simulink model "NarmaMotorS444"  (R2019b)
settings: Solver=FixedStepAuto  StartTime=0.0  StopTime=30  FixedStep=0.001  RelTol=1e-3
libraries: neural x1, simulink x1
settings Model: Creator=Emanuel  LastModifiedBy=Emanuel

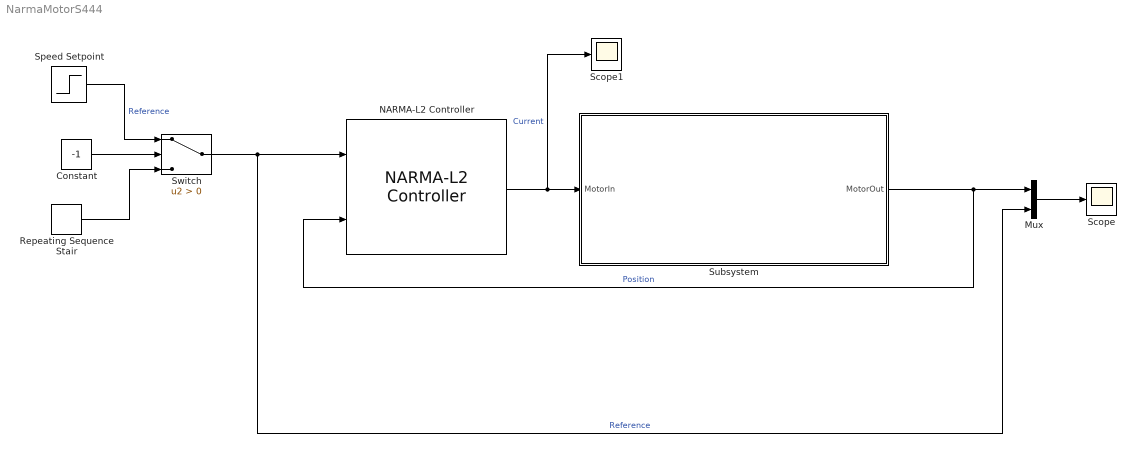
== system NarmaMotorS444 ==
  Constant : Constant  Value=-1
  Mux : Mux  Inputs=2
  NARMA-L2 Controller : neural/Control Systems/NARMA-L2 Controller  Normalize=0  IW1_1=[-0.00010236025899872490809 2.7586514069221412045e-05 -1.0105911937399750936e-05 1.3256012738340794443e-05 -0.00012177307341552546399 9.4877524383052964214e-05 0.00016811599685202734166;-0.9314764402798860754 -4.0881413596783540143 -1.7151050991711540572 4.9130010420420884287 -1.2247909630343454257 -2.4839816062380393191 -2.4615143768260137058;-9.4112593425783597212 6.7702586754591775886 5.1048148087375526671 -4.0293352992265125678 -1.5860815268788490684 -2.0648737785344812856 1.8072837448183800557;-6.6517733281320357008 -0.39174207719143561146 4.2930162877030273449 5.6049907770564697529 -0.78433332140491096585 -0.37768508077910345477 -0.42004150889728419926]  IW3_2=[-1.1884782210932853808 -2.6026502224083305492 0.77838373361354451507 2.7173822538084015932 -0.25745108287285101145 -0.020471196678414908116 -0.46445815351973612772;-0.25444398603368395539 0.30008368263429602285 -0.0074376747696380850552 0.59158184449179707087 0.34380512952139080651 -0.87996185058892895103 1.4365647591299173236;0.077286965668154586351 0.15379022274742931709 0.49370556823373967781 -0.72901144987097687977 -6.3829467961491106465 -24.779081553654108916 7.8291606863920542025;0.60195820662206900309 -2.4802125107952845973 -2.0779594279619324482 4.3693209146217668604 0.97906627286878922245 -0.91348821354353892943 0.52582308602693783595]  IW5_3=2.791472264992422847  LW2_1=[-116.75369921671634188 -15.359712959372973984 -10.101511034971979441 14.81434611829450354]  LW4_3=[-1.5956321863719566956 2.5213572345198809188 2.7013939494135672525 0.99504426028142600735]  LW5_4=-0.13241264861201840208  LW6_5=-3.346419847725022656  LW6_2=119.28421133069207372  B1=[0.47304643530334977708;0.069176646723712875708;-2.1542505763216901471;1.1374465832201940962]  B2=14.49636392954983144  B3=[1.2607629848186907573;0.0297410068321030778;3.2197369295363471586;0.27292507888832240326]  B4=2.1680736346604891907  Limit_output=0  min_output=-Inf  max_output=Inf  Use_Previous_Weights=1  Ts=0.05  S1=4  Ni=4  Nj=4  sim_file=SoleModelNoDistrubance  trainfun=trainlm  Use_validation=1  Use_Testing=1  max_i=40  min_i=1  max_i_int=4  min_i_int=2  sam_training=10000  epochs=500  minp=1.2838861864609374397  maxp=39.753006491435613157  mint=2000.3866487334141766  maxt=39.753006491435613157
      settings: SourceProductName=Deep Learning Toolbox  SourceProductBaseCode=NN
  Repeating Sequence Stair : simulink/Sources/Repeating Sequence Stair  OutValues=[1000 2000 3000 4000 5000].'  tsamp=4  OutMin=[]  OutMax=[]  OutDataTypeStr=double  OutputDataTypeScalingMode=double  OutDataType=fixdt(0,8)  ConRadixGroup=Best Precision: Vector-wise  OutScaling=2^-12
  Scope : Scope
  Scope1 : Scope
  Speed Setpoint : Step  Time=5  Before=2000  After=3000  SampleTime=0
  Subsystem : Subsystem
  Switch : Switch  Criteria=u2 > Threshold
  wires:
  NARMA-L2 Controller/1 -> Scope1/1, Subsystem/1(MotorIn)  "Current"
  Subsystem/1("MotorOut ") -> NARMA-L2 Controller/2, Mux/1  "Position"
  Mux/1 -> Scope/1
  Switch/1 -> Mux/2, NARMA-L2 Controller/1  "Reference"
  Repeating Sequence Stair/1 -> Switch/3
  Speed Setpoint/1 -> Switch/1  "Reference"
  Constant/1 -> Switch/2

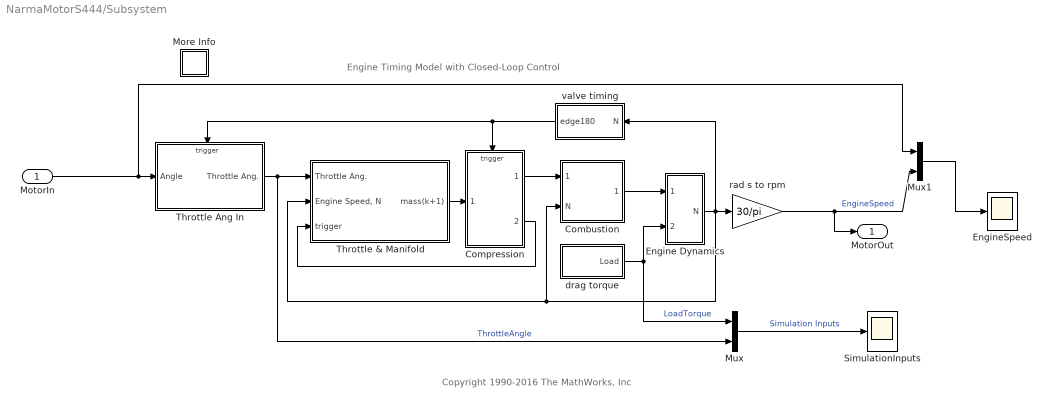
== system NarmaMotorS444/Subsystem ==
  note: Copyright 1990-2016 The MathWorks, Inc
  note: Engine Timing Model with Closed-Loop Control
  MotorIn : Inport
  Combustion : Subsystem
  Compression : Subsystem  TreatAsAtomicUnit=on
  Engine Dynamics : Subsystem
  EngineSpeed : Scope
  More Info : Subsystem
      settings: OpenFcn=showdemo(bdroot(gcb))
      mask Display: disp('?')
  Mux : Mux  Inputs=2
  Mux1 : Mux  Inputs=2
  SimulationInputs : Scope
  Throttle & Manifold : Subsystem
  Throttle Ang In : Subsystem  TreatAsAtomicUnit=on
  drag torque : Subsystem
  rad s to rpm : Gain  Gain=30/pi  SaturateOnIntegerOverflow=on  OutDataTypeStr=Inherit: Same as input  ParamDataTypeStr=Inherit: Same as input
  valve timing : Subsystem
  "MotorOut " : Outport
  wires:
  Combustion/1(Torque) -> Engine Dynamics/1(Teng)
  Throttle Ang In/1(Throttle Ang.) -> Mux/2, Throttle & Manifold/1(Throttle Ang.)  "ThrottleAngle"
  drag torque/1(Load) -> Mux/1, Engine Dynamics/2(Tload)  "LoadTorque"
  MotorIn/1 -> Mux1/1, Throttle Ang In/1(Angle)
  Throttle & Manifold/1(mass(k+1)) -> Compression/1(mass(k+1))
  Compression/2(trigger) -> Throttle & Manifold/3(trigger)
  Mux/1 -> SimulationInputs/1  "Simulation Inputs"
  rad s to rpm/1 -> "MotorOut "/1, Mux1/2  "EngineSpeed"
  Compression/1(mass(k)) -> Combustion/1(Air Charge)
  Mux1/1 -> EngineSpeed/1
  valve timing/1(edge180) -> Throttle Ang In/Trigger, Compression/Trigger
  Engine Dynamics/1(N) -> rad s to rpm/1, valve timing/1(N), Throttle & Manifold/2("Engine Speed, N"), Combustion/2(N)

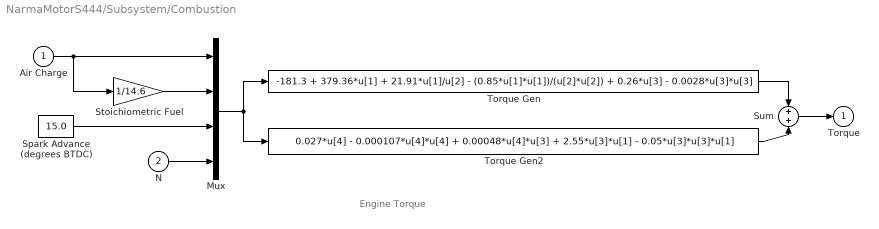
== system NarmaMotorS444/Subsystem/Combustion ==
  note: Engine Torque
  Air Charge : Inport
  N : Inport  Port=2
  Mux : Mux
  Spark Advance (degrees BTDC) : Constant  Value=15.0
  Stoichiometric Fuel : Gain  Gain=1/14.6  SaturateOnIntegerOverflow=on  OutDataTypeStr=Inherit: Same as input  ParamDataTypeStr=Inherit: Same as input
  Sum : Sum  SaturateOnIntegerOverflow=on  InputSameDT=on  OutDataTypeStr=Inherit: Same as first input
  Torque Gen : Fcn  Expr=-181.3 + 379.36*u[1] + 21.91*u[1]/u[2] - (0.85*u[1]*u[1])/(u[2]*u[2]) + 0.26*u[3] - 0.0028*u[3]*u[3]
  Torque Gen2 : Fcn  Expr=0.027*u[4] - 0.000107*u[4]*u[4] + 0.00048*u[4]*u[3] + 2.55*u[3]*u[1] - 0.05*u[3]*u[3]*u[1]
  Torque : Outport  InitialOutput=0
  wires:
  Stoichiometric Fuel/1 -> Mux/2
  Spark Advance (degrees BTDC)/1 -> Mux/3
  N/1 -> Mux/4
  Air Charge/1 -> Stoichiometric Fuel/1, Mux/1
  Mux/1 -> Torque Gen/1, Torque Gen2/1
  Torque Gen2/1 -> Sum/2
  Torque Gen/1 -> Sum/1
  Sum/1 -> Torque/1

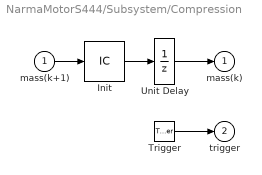
== system NarmaMotorS444/Subsystem/Compression ==
  mass(k+1) : Inport
  Trigger : TriggerPort  TriggerType=either  VariantControl=Variant  ShowOutputPort=on
  Init : InitialCondition  Value=0.152
  Unit Delay : UnitDelay  InitialCondition=0.152  SampleTime=-1  HasFrameUpgradeWarning=on
  mass(k) : Outport  InitialOutput=0.152
  trigger : Outport  Port=2  InitialOutput=-1
  wires:
  Init/1 -> Unit Delay/1
  mass(k+1)/1 -> Init/1
  Unit Delay/1 -> mass(k)/1
  Trigger/1 -> trigger/1

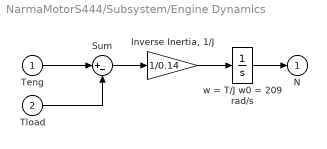
== system NarmaMotorS444/Subsystem/Engine Dynamics ==
  Teng : Inport
  Tload : Inport  Port=2
  "Inverse Inertia, 1/J" : Gain  Gain=1/0.14  SaturateOnIntegerOverflow=on  OutDataTypeStr=Inherit: Same as input  ParamDataTypeStr=Inherit: Same as input
  Sum : Sum  Inputs=|+-  SaturateOnIntegerOverflow=on  InputSameDT=on  OutDataTypeStr=Inherit: Same as first input
  w = T/J w0 = 209 rad/s : Integrator  InitialCondition=209.48
  N : Outport  InitialOutput=0
  wires:
  "Inverse Inertia, 1/J"/1 -> w = T/J w0 = 209 rad/s/1
  w = T/J w0 = 209 rad/s/1 -> N/1
  Sum/1 -> "Inverse Inertia, 1/J"/1
  Teng/1 -> Sum/1
  Tload/1 -> Sum/2

== system NarmaMotorS444/Subsystem/More Info ==

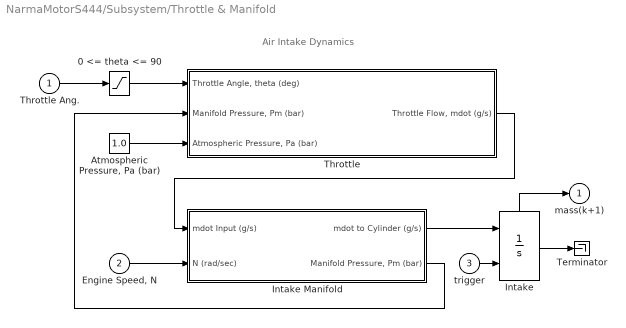
== system NarmaMotorS444/Subsystem/Throttle & Manifold ==
  note: Air Intake Dynamics
  Throttle Ang. : Inport
  "Engine Speed, N" : Inport  Port=2
  trigger : Inport  Port=3
  0 <= theta <= 90 : Saturate  UpperLimit=90  LowerLimit=0
  "Atmospheric Pressure, Pa (bar)" : Constant  Value=1.0
  Intake : Integrator  ExternalReset=either  ShowStatePort=on
  Intake Manifold : Subsystem
  Terminator : Terminator
  Throttle : Subsystem
  mass(k+1) : Outport  InitialOutput=0
  wires:
  0 <= theta <= 90/1 -> Throttle/1("Throttle Angle, theta (deg)")
  Throttle Ang./1 -> 0 <= theta <= 90/1
  Throttle/1("Throttle Flow, mdot (g/s)") -> Intake Manifold/1(mdot Input (g/s))
  "Engine Speed, N"/1 -> Intake Manifold/2(N (rad/sec))
  Intake Manifold/2("Manifold Pressure, Pm (bar)") -> Throttle/2("Manifold Pressure, Pm (bar)")
  Intake Manifold/1(mdot to Cylinder (g/s)) -> Intake/1
  "Atmospheric Pressure, Pa (bar)"/1 -> Throttle/3("Atmospheric Pressure, Pa (bar) ")
  Intake/State -> mass(k+1)/1
  trigger/1 -> Intake/2
  Intake/1 -> Terminator/1

== system NarmaMotorS444/Subsystem/Throttle Ang In ==
  note: Controller Subsystem
  Angle : Inport
  Trigger : TriggerPort  TriggerType=either  VariantControl=Variant
  Throttle Ang. : Outport  InitialOutput=8.973
  wires:
  Angle/1 -> Throttle Ang./1

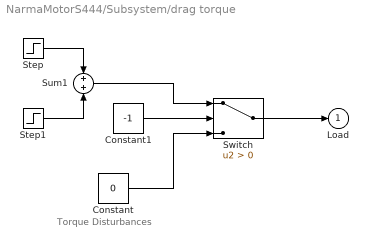
== system NarmaMotorS444/Subsystem/drag torque ==
  note: Torque Disturbances
  Constant : Constant  Value=0
  Constant1 : Constant  Value=-1
  Step : Step  Time=2  Before=25  After=20  SampleTime=0
  Step1 : Step  Time=8  After=5  SampleTime=0
  Sum1 : Sum  SaturateOnIntegerOverflow=on  InputSameDT=on  OutDataTypeStr=Inherit: Same as first input
  Switch : Switch  Criteria=u2 > Threshold
  Load : Outport  InitialOutput=0
  wires:
  Sum1/1 -> Switch/1
  Step/1 -> Sum1/1
  Step1/1 -> Sum1/2
  Switch/1 -> Load/1
  Constant/1 -> Switch/3
  Constant1/1 -> Switch/2

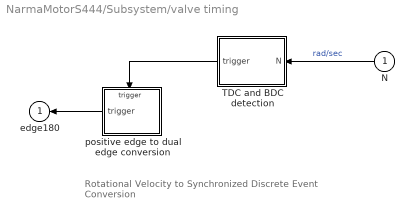
== system NarmaMotorS444/Subsystem/valve timing ==
  note: Rotational Velocity to Synchronized
      | Discrete Event Conversion
  N : Inport
  TDC and BDC detection : Subsystem
  positive edge to dual edge conversion : Subsystem  TreatAsAtomicUnit=on
  edge180 : Outport  InitialOutput=-1
  wires:
  TDC and BDC detection/1(trigger) -> positive edge to dual edge conversion/Trigger
  positive edge to dual edge conversion/1(trigger) -> edge180/1
  N/1 -> TDC and BDC detection/1(N)  "rad/sec"

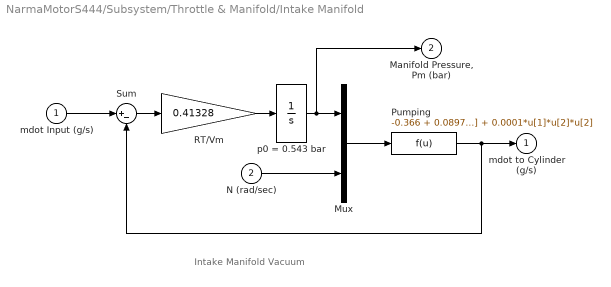
== system NarmaMotorS444/Subsystem/Throttle & Manifold/Intake Manifold ==
  note: Intake Manifold Vacuum
  mdot Input (g/s) : Inport
  N (rad/sec) : Inport  Port=2
  Mux : Mux  Inputs=2
  Pumping : Fcn  Expr=-0.366 + 0.08979*u[1]*u[2] - 0.0337*u[2]*u[1]*u[1] + 0.0001*u[1]*u[2]*u[2]
  RT/Vm : Gain  Gain=0.41328  SaturateOnIntegerOverflow=on  OutDataTypeStr=Inherit: Same as input  ParamDataTypeStr=Inherit: Same as input
  Sum : Sum  Inputs=|+-  SaturateOnIntegerOverflow=on  InputSameDT=on  OutDataTypeStr=Inherit: Same as first input
  p0 = 0.543 bar : Integrator  InitialCondition=.543
  mdot to Cylinder (g/s) : Outport  InitialOutput=0
  "Manifold Pressure, Pm (bar)" : Outport  Port=2  InitialOutput=0
  wires:
  mdot Input (g/s)/1 -> Sum/1
  RT/Vm/1 -> p0 = 0.543 bar/1
  N (rad/sec)/1 -> Mux/2
  Mux/1 -> Pumping/1
  p0 = 0.543 bar/1 -> Mux/1, "Manifold Pressure, Pm (bar)"/1
  Sum/1 -> RT/Vm/1
  Pumping/1 -> Sum/2, mdot to Cylinder (g/s)/1

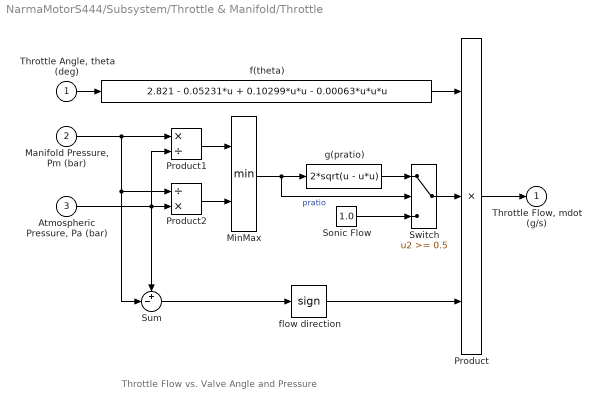
== system NarmaMotorS444/Subsystem/Throttle & Manifold/Throttle ==
  note: Throttle Flow vs. Valve Angle and Pressure
  "Throttle Angle, theta (deg)" : Inport
  "Manifold Pressure, Pm (bar)" : Inport  Port=2
  "Atmospheric Pressure, Pa (bar) " : Inport  Port=3
  MinMax : MinMax  Inputs=2  SaturateOnIntegerOverflow=on  InputSameDT=on
  Product : Product  Inputs=3  SaturateOnIntegerOverflow=on  RndMeth=Zero  InputSameDT=on  OutDataTypeStr=Inherit: Same as first input
  Product1 : Product  Inputs=*/  SaturateOnIntegerOverflow=on  RndMeth=Zero  InputSameDT=on  OutDataTypeStr=Inherit: Same as first input
  Product2 : Product  Inputs=/*  SaturateOnIntegerOverflow=on  RndMeth=Zero  InputSameDT=on  OutDataTypeStr=Inherit: Same as first input
  "Sonic Flow " : Constant  Value=1.0
  Sum : Sum  Inputs=+-|  SaturateOnIntegerOverflow=on  InputSameDT=on  OutDataTypeStr=Inherit: Same as first input
  Switch : Switch  Threshold=0.5  SaturateOnIntegerOverflow=on  InputSameDT=on
  f(theta) : Fcn  Expr=2.821 - 0.05231*u + 0.10299*u*u - 0.00063*u*u*u
  flow direction : Signum
  g(pratio) : Fcn  Expr=2*sqrt(u - u*u)
  "Throttle Flow, mdot (g/s)" : Outport  InitialOutput=0
  wires:
  "Manifold Pressure, Pm (bar)"/1 -> Sum/2, Product2/1, Product1/1
  Product2/1 -> MinMax/2
  Product1/1 -> MinMax/1
  "Atmospheric Pressure, Pa (bar) "/1 -> Sum/1, Product2/2, Product1/2
  g(pratio)/1 -> Switch/1
  "Sonic Flow "/1 -> Switch/3
  Switch/1 -> Product/2
  flow direction/1 -> Product/3
  Sum/1 -> flow direction/1
  MinMax/1 -> Switch/2, g(pratio)/1  "pratio"
  "Throttle Angle, theta (deg)"/1 -> f(theta)/1
  Product/1 -> "Throttle Flow, mdot (g/s)"/1
  f(theta)/1 -> Product/1

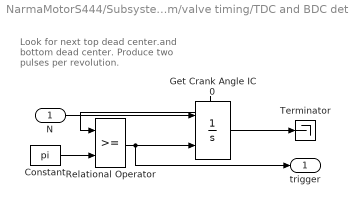
== system NarmaMotorS444/Subsystem/valve timing/TDC and BDC detection ==
  note: Look for next top dead center.and
      | bottom dead center.
      | Produce two pulses per revolution.
  N : Inport
  Constant : Constant  Value=pi
  Get Crank Angle IC 0 : Integrator  ExternalReset=rising  ShowStatePort=on
  Relational Operator : RelationalOperator  OutDataTypeStr=boolean  RndMeth=Nearest  InputSameDT=on
  Terminator : Terminator
  trigger : Outport  InitialOutput=0
  wires:
  N/1 -> Get Crank Angle IC 0/1
  Relational Operator/1 -> trigger/1, Get Crank Angle IC 0/2
  Constant/1 -> Relational Operator/2
  Get Crank Angle IC 0/State -> Relational Operator/1
  Get Crank Angle IC 0/1 -> Terminator/1

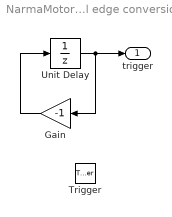
== system NarmaMotorS444/Subsystem/valve timing/positive edge to dual edge conversion ==
  Trigger : TriggerPort  VariantControl=Variant
  Gain : Gain  Gain=-1  SaturateOnIntegerOverflow=on  OutDataTypeStr=Inherit: Same as input  ParamDataTypeStr=Inherit: Same as input
  Unit Delay : UnitDelay  InitialCondition=1  SampleTime=-1  HasFrameUpgradeWarning=on
  trigger : Outport  InitialOutput=-1
  wires:
  Gain/1 -> Unit Delay/1
  Unit Delay/1 -> trigger/1, Gain/1
